simulink model "sim12ex9"  (Simulink 4.00)
settings: Solver=ode23  SolverMode=SingleTasking  StartTime=0.0  StopTime=15  MaxStep=.05  RelTol=1e-3  AbsTol=1e-3
libraries: simulink_extras x1
settings Model: LastModifiedBy=saadat  SaveTime=off  SaveOutput=off  LimitDataPoints=off  RTWTemplateMakefile=grt_vc.tmf  ExtModeTrigMode=oneshot  ExtModeArmWhenConnect=off

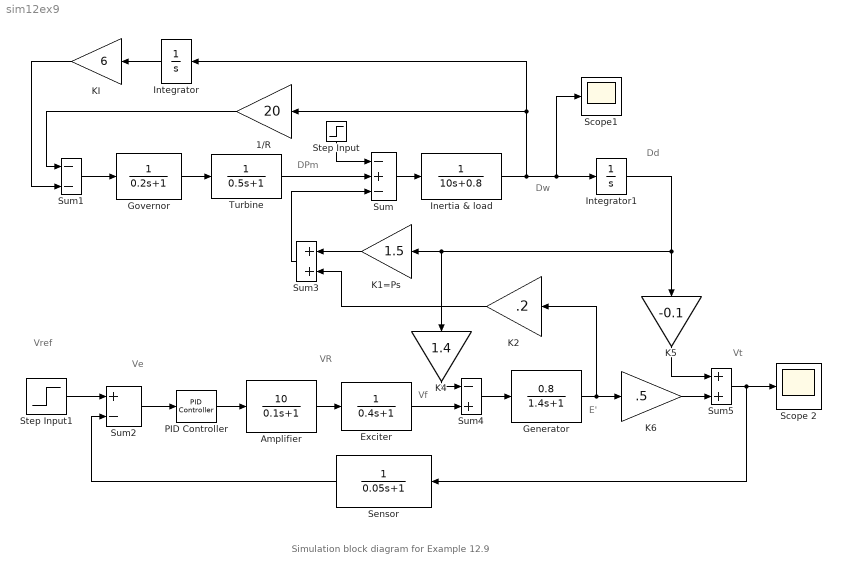
== system sim12ex9 ==
  note: Simulation block diagram for Example 12.9
  note: Dw
  note: Dd
  note: Vf
  note: VR
  note: E'
  note: Vt
  note: Ve
  note: Vref
  note: DPm
  1/R : Gain  Orientation=left  Gain=20  Multiplication=Element-wise(K.*u)  SaturateOnIntegerOverflow=on
  Amplifier : TransferFcn  Numerator=10  Denominator="[0.1  1]"  AbsoluteTolerance=auto  Realization=auto
  Exciter : TransferFcn  Numerator=1  Denominator="[0.4  1]"  AbsoluteTolerance=auto  Realization=auto
  Generator : TransferFcn  Numerator=[0.8]  Denominator=[ 1.4 1]  AbsoluteTolerance=auto  Realization=auto
  Governor : TransferFcn  Numerator=[1]  Denominator="[0.2   1]"  AbsoluteTolerance=auto  Realization=auto
  Inertia & load : TransferFcn  Numerator=[1]  Denominator="[10  0.8]"  AbsoluteTolerance=auto  Realization=auto
  Integrator : Integrator  Orientation=left  ExternalReset=none  InitialConditionSource=internal  InitialCondition=0  LimitOutput=off  UpperSaturationLimit=inf  LowerSaturationLimit=-inf  ShowSaturationPort=off  ShowStatePort=off  AbsoluteTolerance=auto
  Integrator1 : Integrator  ExternalReset=none  InitialConditionSource=internal  InitialCondition=0  LimitOutput=off  UpperSaturationLimit=inf  LowerSaturationLimit=-inf  ShowSaturationPort=off  ShowStatePort=off  AbsoluteTolerance=auto
  K1=Ps : Gain  Orientation=left  Gain=1.5  Multiplication=Element-wise(K.*u)  SaturateOnIntegerOverflow=on
  K2 : Gain  Orientation=left  Gain=.2  Multiplication=Element-wise(K.*u)  SaturateOnIntegerOverflow=on
  K4 : Gain  Orientation=down  Gain=1.4  Multiplication=Element-wise(K.*u)  SaturateOnIntegerOverflow=on
  K5 : Gain  Orientation=down  Gain=-0.1  Multiplication=Element-wise(K.*u)  SaturateOnIntegerOverflow=on
  K6 : Gain  Gain=.5  Multiplication=Element-wise(K.*u)  SaturateOnIntegerOverflow=on
  KI : Gain  Orientation=left  Gain=6  Multiplication=Element-wise(K.*u)  SaturateOnIntegerOverflow=on
  PID Controller : simulink_extras/Additional Linear/PID Controller  P=1  I=0.25  D=0.3
  Scope 2 : Scope
      settings: TickLabels=on  TimeRange=15  YMin=0  YMax=1  SaveToWorkspace=off  SaveName=ScopeData  DataFormat=Array  LimitDataPoints=on  MaxDataPoints=5000
  Scope1 : Scope
      settings: TickLabels=on  TimeRange=15  YMin=-0.04  YMax=0.01  SaveToWorkspace=off  SaveName=ScopeData  DataFormat=Array  LimitDataPoints=on  MaxDataPoints=5000
  Sensor : TransferFcn  Orientation=left  Numerator=[1]  Denominator="[0.05  1]"  AbsoluteTolerance=auto  Realization=auto
  Step Input : Step  Orientation=down  Time=0  Before=0  After=0.2  SampleTime=0
  Step Input1 : Step  Time=0  Before=0  After=1  SampleTime=0
  Sum : Sum  Inputs=-+-  SaturateOnIntegerOverflow=on
  Sum1 : Sum  Inputs=--  SaturateOnIntegerOverflow=on
  Sum2 : Sum  Inputs=+-  SaturateOnIntegerOverflow=on
  Sum3 : Sum  Orientation=left  Inputs=++  SaturateOnIntegerOverflow=on
  Sum4 : Sum  Inputs=-+  SaturateOnIntegerOverflow=on
  Sum5 : Sum  Inputs=++  SaturateOnIntegerOverflow=on
  Turbine : TransferFcn  Numerator=[1]  Denominator="[0.5  1]"  AbsoluteTolerance=auto  Realization=auto
  wires:
  Inertia & load/1 -> 1/R/1, Integrator/1, Scope1/1, Integrator1/1
  Integrator1/1 -> K4/1, K1=Ps/1, K5/1
  KI/1 -> Sum1/2
  Integrator/1 -> KI/1
  1/R/1 -> Sum1/1
  K2/1 -> Sum3/2
  K4/1 -> Sum4/1
  Generator/1 -> K2/1, K6/1
  Sum5/1 -> Sensor/1, Scope 2/1
  K5/1 -> Sum5/1
  K1=Ps/1 -> Sum3/1
  K6/1 -> Sum5/2
  Sum4/1 -> Generator/1
  Exciter/1 -> Sum4/2
  Sum3/1 -> Sum/3
  PID Controller/1 -> Amplifier/1
  Sum2/1 -> PID Controller/1
  Amplifier/1 -> Exciter/1
  Sensor/1 -> Sum2/2
  Step Input1/1 -> Sum2/1
  Step Input/1 -> Sum/1
  Sum1/1 -> Governor/1
  Sum/1 -> Inertia & load/1
  Turbine/1 -> Sum/2
  Governor/1 -> Turbine/1
